simulink model "HighTemperatureOven_KalmanFilter_Simulink2019b"  (R2020b)
settings: Solver=ode4  StartTime=0.0  StopTime=SIM_TIME  FixedStep=STEP_SIZE  RelTol=1e-3
undefined symbols (not defined in the file): C_kf, Cg, Cs, F_kf, G_kf, k, kc, kg, kr, L_kf, STEP_SIZE, t_step_Ta, Ta0K, TafK, Tg0K, Ts0K, Tsampl, u0, umax, umin, V2d, x0hat, yss
libraries: simulink x1
settings Model: Creator=Mikkel  LastModifiedBy=roga
settings DataIOCC: LimitDataPoints=on  SaveFormat=Array  ReturnWorkspaceOutputs=off
settings OptimizationCC: ExpressionDepthLimit=2147483647  LifeSpan=inf
settings DebuggingCC: UnderspecifiedInitializationDetection=Classic  MergeDetectMultiDrivingBlocksExec=none  SolverPrmCheckMsg=warning  FcnCallInpInsideContextMsg=warning  StateNameClashWarn=warning  SFUnexpectedBacktrackingDiag=warning  SFNoUnconditionalDefaultTransitionDiag=warning  SFExecutionAtInitializationDiag=none  ArithmeticOperatorsInVariantConditions=warning
settings HardwareCC: ProdBitPerPointer=32  ProdBitPerSizeT=32  ProdBitPerPtrDiffT=32  ProdLargestAtomicFloat=None  ProdIntDivRoundTo=Undefined  ProdEndianess=Unspecified  ProdWordSize=32  ProdHWDeviceType=32-bit Generic
settings ModelReferenceCC: PropagateSignalLabelsOutOfModel=off
settings SFSimCC: SimUseLocalCustomCode=off  CustomCodeUndefinedFunction=UseInterfaceOnly
settings RTWCC: RTWUseLocalCustomCode=off
settings CodeAppCC: StateflowObjectComments=on
settings GRTTargetCC: TargetLangStandard=C89/C90 (ANSI)  CombineOutputUpdateFcns=off  GRTInterface=on
settings ConfigComp: CovMetricSettings=dw  CovSaveCumulativeToWorkspaceVar=on  CovSaveSingleToWorkspaceVar=on  CovExternalEMLEnable=off  CovSFcnEnable=off

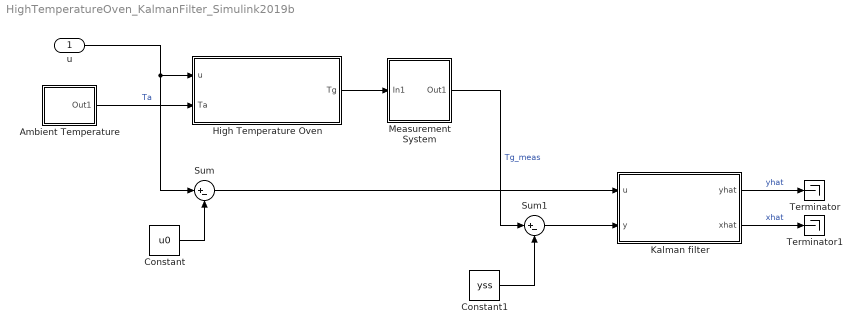
== system HighTemperatureOven_KalmanFilter_Simulink2019b ==
  u : Inport
  Ambient Temperature : Subsystem
  Constant : Constant  Value=u0  SampleTime=Tsampl
  Constant1 : Constant  Value=yss  SampleTime=Tsampl
  High Temperature Oven : Subsystem
  Kalman filter : Subsystem
  Measurement System : Subsystem
  Sum : Sum  Inputs=|+-
  Sum1 : Sum  Inputs=|+-
  Terminator : Terminator
  Terminator1 : Terminator
  wires:
  u/1 -> Sum/1, High Temperature Oven/1(u)
  High Temperature Oven/1(Tg) -> Measurement System/1(In1)
  Kalman filter/1(yhat) -> Terminator/1  "yhat"
  Kalman filter/2(xhat) -> Terminator1/1  "xhat"
  Ambient Temperature/1(Out1) -> High Temperature Oven/2(Ta)  "Ta"
  Sum/1 -> Kalman filter/1(u)
  Sum1/1 -> Kalman filter/2(y)
  Measurement System/1(Out1) -> Sum1/1  "Tg_meas"
  Constant/1 -> Sum/2
  Constant1/1 -> Sum1/2

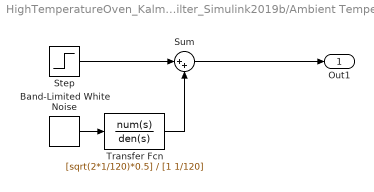
== system HighTemperatureOven_KalmanFilter_Simulink2019b/Ambient Temperature ==
  Band-Limited White Noise : simulink/Sources/Band-Limited White Noise  Cov=1  Ts=STEP_SIZE  seed=[23341]
  Step : Step  Time=t_step_Ta  Before=Ta0K  After=TafK  SampleTime=0
  Sum : Sum  Inputs=|++
  Transfer Fcn : TransferFcn  Numerator=[sqrt(2*1/120)*0.5]  Denominator=[1 1/120]
  Out1 : Outport
  wires:
  Transfer Fcn/1 -> Sum/2
  Band-Limited White Noise/1 -> Transfer Fcn/1
  Sum/1 -> Out1/1
  Step/1 -> Sum/1

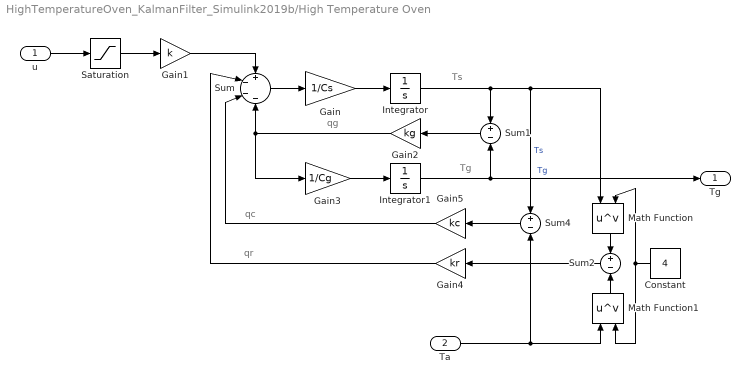
== system HighTemperatureOven_KalmanFilter_Simulink2019b/High Temperature Oven ==
  note: qg
  note: Ts
  note: Tg
  note: qr
  note: qc
  u : Inport
  Ta : Inport  Port=2
  Constant : Constant  Value=4
  Gain : Gain  Gain=1/Cs
  Gain1 : Gain  Gain=k
  Gain2 : Gain  Gain=kg
  Gain3 : Gain  Gain=1/Cg
  Gain4 : Gain  Gain=kr
  Gain5 : Gain  Gain=kc
  Integrator : Integrator  Priority=1  InitialCondition=Ts0K
  Integrator1 : Integrator  Priority=2  InitialCondition=Tg0K
  Math Function : Math  Operator=pow  SignedPower=on  SaturateOnIntegerOverflow=on
  Math Function1 : Math  Operator=pow  SignedPower=on  SaturateOnIntegerOverflow=on
  Saturation : Saturate  UpperLimit=umax  LowerLimit=umin
  Sum : Sum  Inputs=+---
  Sum1 : Sum  Inputs=+-
  Sum2 : Sum  Inputs=+-
  Sum4 : Sum  Inputs=+-
  Tg : Outport
  wires:
  Sum/1 -> Gain/1
  Integrator/1 -> Sum1/1, Sum4/1, Math Function/1  "Ts"
  Ta/1 -> Math Function1/1, Sum4/2
  Gain4/1 -> Sum/2
  Integrator1/1 -> Tg/1, Sum1/2  "Tg"
  Sum2/1 -> Gain4/1
  Gain1/1 -> Sum/1
  Constant/1 -> Math Function/2, Math Function1/2
  Gain/1 -> Integrator/1
  Gain2/1 -> Gain3/1, Sum/4
  Sum1/1 -> Gain2/1
  Math Function1/1 -> Sum2/2
  Math Function/1 -> Sum2/1
  Gain3/1 -> Integrator1/1
  Sum4/1 -> Gain5/1
  Gain5/1 -> Sum/3
  u/1 -> Saturation/1
  Saturation/1 -> Gain1/1

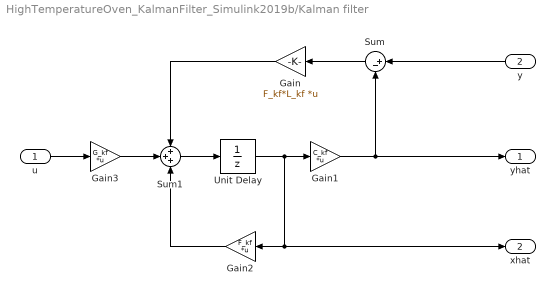
== system HighTemperatureOven_KalmanFilter_Simulink2019b/Kalman filter ==
  u : Inport
  y : Inport  Port=2
  Gain : Gain  Gain=F_kf*L_kf  Multiplication=Matrix(K*u) (u vector)
  Gain1 : Gain  Gain=C_kf  Multiplication=Matrix(K*u) (u vector)
  Gain2 : Gain  Gain=F_kf  Multiplication=Matrix(K*u) (u vector)
  Gain3 : Gain  Gain=G_kf  Multiplication=Matrix(K*u) (u vector)
  Sum : Sum  Inputs=|+-
  Sum1 : Sum  Inputs=+++
  Unit Delay : UnitDelay  InitialCondition=x0hat  SampleTime=Tsampl  HasFrameUpgradeWarning=on
  yhat : Outport  VectorParamsAs1DForOutWhenUnconnected=off
  xhat : Outport  Port=2  VectorParamsAs1DForOutWhenUnconnected=off
  wires:
  Gain3/1 -> Sum1/2
  y/1 -> Sum/1
  Gain/1 -> Sum1/1
  Sum/1 -> Gain/1
  u/1 -> Gain3/1
  Gain2/1 -> Sum1/3
  Sum1/1 -> Unit Delay/1
  Gain1/1 -> yhat/1, Sum/2
  Unit Delay/1 -> xhat/1, Gain2/1, Gain1/1

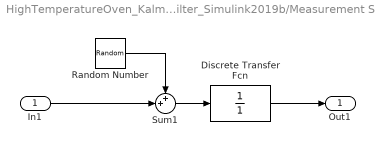
== system HighTemperatureOven_KalmanFilter_Simulink2019b/Measurement System ==
  In1 : Inport
  Discrete Transfer Fcn : DiscreteTransferFcn  Denominator=[1]  SampleTime=Tsampl
  Random Number : RandomNumber  Variance=V2d  SampleTime=Tsampl
  Sum1 : Sum  Inputs=++|
  Out1 : Outport
  wires:
  Random Number/1 -> Sum1/1
  In1/1 -> Sum1/2
  Sum1/1 -> Discrete Transfer Fcn/1
  Discrete Transfer Fcn/1 -> Out1/1
